simulink model "Solar"  (R2024b)
settings: Solver=VariableStepAuto  StartTime=0.0  StopTime=10.0  RelTol=1e-3
undefined symbols (not defined in the file): sigbuilder_block
libraries: spsSeriesRLCBranchLib x9, spsVoltageMeasurementLib x8, spsDiodeLib x4, spsIGBTLib x1, spsPVArrayLib x1, spsCurrentMeasurementLib x1, spsMosfetLib x1, spsPWMGeneratorDCDCLib x1, sps_lib x1
settings Model: SimulationMode=accelerator  Creator=Jatay  LastModifiedBy=Jatay

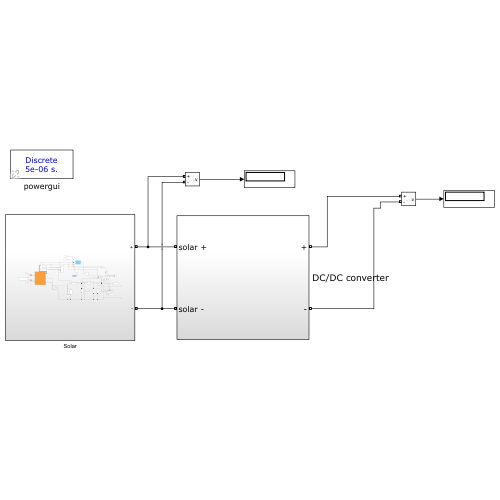
[thumbnail: Simulink's stored preview of the top-level diagram]
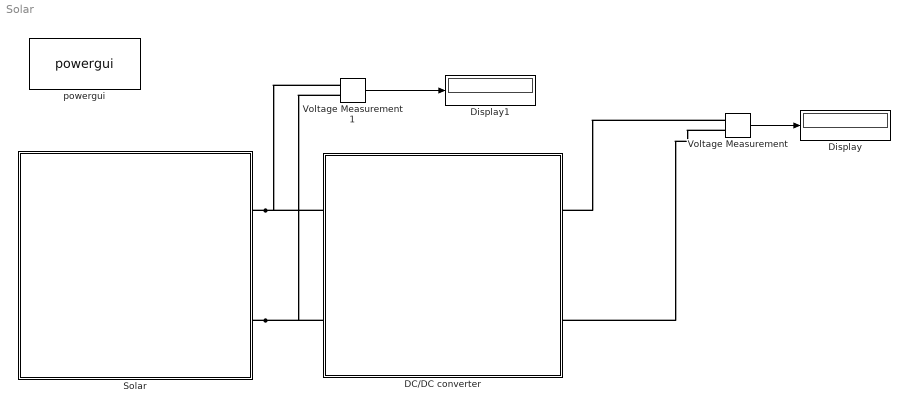
== system Solar ==
  DC/DC converter : Subsystem
  Display : Display
  Display1 : Display
  Solar : Subsystem
  Voltage Measurement : spsVoltageMeasurementLib/Voltage Measurement  PhasorSimulation=off  OutputType=Complex  PSBequivalent=0
  Voltage Measurement1 : spsVoltageMeasurementLib/Voltage Measurement  PhasorSimulation=off  OutputType=Complex  PSBequivalent=0
  powergui : sps_lib/powergui  Priority=1  SimulationMode=Discrete  SampleTime=5e-6  frequency=60  Iterations=50  frequencyindice=0  Pbase=100e6  ErrMax=1e-4  UnitsV=kV  UnitsW=MW  buscounter=0  FunctionMessages=off  echomessages=off  EnableUseOfTLC=off  CurrentSourceSwitches=off  DisableSnubberDevices=off  DisableRonSwitches=off  DisableVfSwitches=off  DisplayEquations=off  AutomaticDiscreteSolvers=off  SolverType=Tustin  Interpol=off  ExternalGateDelay=off  methode=off  Ts=0  x0status=blocks  SPID=off  SwTol=0  HookPort=off  NonlinearTolerance=1e-4  nMaxIteration=100  ContinueOnMaxIteration=off  RestoreLinks=warning  ResistiveCurrentMeasurement=off  Frange=[0:2:500]  Ylog=off  Xlog=on  ShowGrid=off  save=off  variable=ZData  structure=0  ZoomFFT=off  StartTime=0.0  cycles=1  DisplayStyle=1  fundamental=60  FreqAxis=off  MaxFrequency=1000  frequencyindicesteady=1  RmsSteady=1  display=off
  wires:
  Voltage Measurement1/1 -> Display1/1
  Voltage Measurement/1 -> Display/1
  connections:
  Solar/RConn1 -- DC/DC converter/LConn1 -- Voltage Measurement1/LConn1
  Solar/RConn2 -- DC/DC converter/LConn2 -- Voltage Measurement1/LConn2
  Voltage Measurement/LConn2 -- DC/DC converter/RConn2
  Voltage Measurement/LConn1 -- DC/DC converter/RConn1

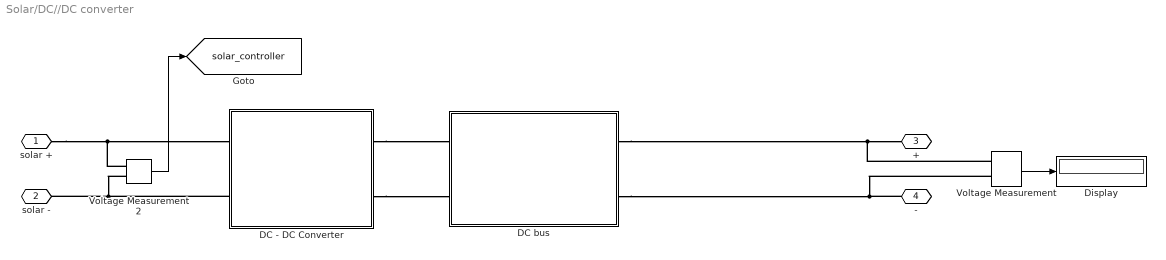
== system Solar/DC//DC converter ==
  DC - DC Converter : Subsystem
  DC bus : Subsystem
  Display : Display
  Voltage Measurement : spsVoltageMeasurementLib/Voltage Measurement  PhasorSimulation=off  OutputType=Complex  PSBequivalent=0
  Voltage Measurement2 : spsVoltageMeasurementLib/Voltage Measurement  PhasorSimulation=off  OutputType=Complex  PSBequivalent=0
  solar + : PMIOPort  Side=Left
  solar - : PMIOPort  Port=2  Side=Left
  + : PMIOPort  Port=3  Side=Right
  - : PMIOPort  Port=4  Side=Right
  tag scope: solar_controller=global
  wires:
  Voltage Measurement2/1 -> [solar_controller]
  Voltage Measurement/1 -> Display/1
  connections:
  DC - DC Converter/RConn1 -- DC bus/LConn1
  solar +/RConn1 -- DC - DC Converter/LConn1 -- Voltage Measurement2/LConn1
  DC - DC Converter/LConn2 -- Voltage Measurement2/LConn2 -- solar -/RConn1
  DC - DC Converter/RConn2 -- DC bus/LConn2
  -/RConn1 -- DC bus/RConn2 -- Voltage Measurement/LConn2
  Voltage Measurement/LConn1 -- DC bus/RConn1 -- +/RConn1

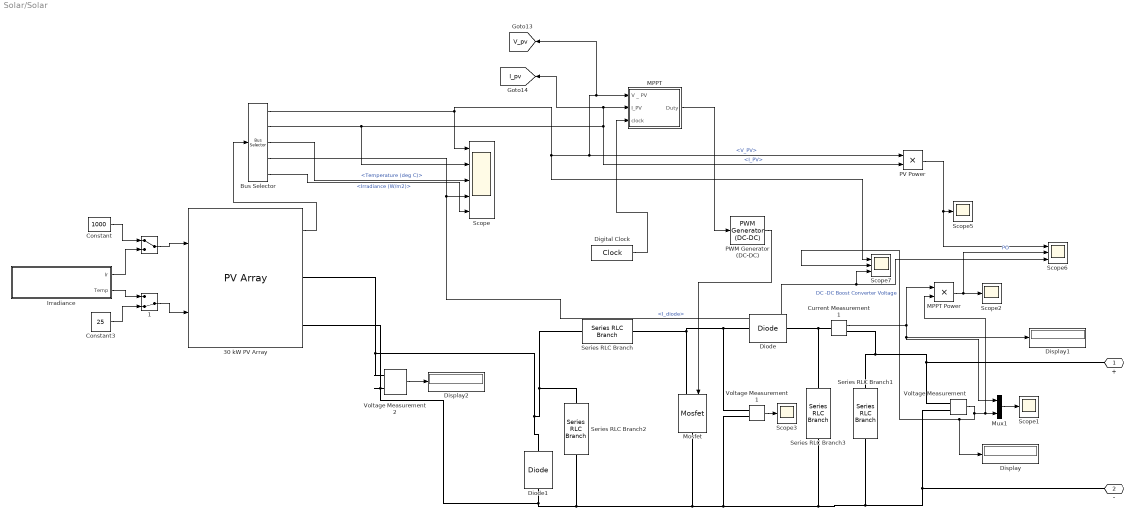
== system Solar/Solar ==
  "      " : ManualSwitch
  "      1" : ManualSwitch  CurrentSetting=0
  30 kW PV Array : spsPVArrayLib/PV Array  Npar=15  Nser=10  PlotType=array @ 1000 W/m2 & specified temperatures  S_vec="[ 1000  500  100 ]"  Temp_C_vec="[ 45 25  ]"  ModuleName=User-defined  PlotWhenSelected=off  Pm=213.15  Ncell=60  Voc=48  Isc=7.84  Vm=29  Im=7.35  beta_Voc_pc=-0.36099  alpha_Isc_pc=0.102  beta_Voc=-0.17328  alpha_Isc=0.0079968  IL=8.2285  I0=2.9956e-10  nI=1.2955  Rsh=7353.5939  Rs=2.0228  RobustModel=off  RobustCellTemperature=25  BAL=on  Tc=1e-6  Tfilter=5e-5
  Bus Selector : BusSelector  OutputSignals=V_PV,I_PV,Temperature (deg C),I_diode,Irradiance (W/m2)
  Constant : Constant  Value=1000
  Constant3 : Constant  Value=25
  Current Measurement1 : spsCurrentMeasurementLib/Current Measurement  PhasorSimulation=off  OutputType=Complex  PSBequivalent=0
  Digital Clock : DigitalClock  SampleTime=0.001
  Diode : spsDiodeLib/Diode  Ron=0.5  Lon=0  Vf=0.7  IC=0  UseSnubber=0  Rs=1e5  Cs=250e-9  Measurements=off
  Diode1 : spsDiodeLib/Diode  Ron=0.5  Lon=0  Vf=0.7  IC=0  UseSnubber=0  Rs=1e5  Cs=250e-9  Measurements=off
  Display : Display
  Display1 : Display
  Display2 : Display
  "Irradiance " : Subsystem  Tag=STV Subsys  LoadFcn=sigbuilder_block('load');  StartFcn=sigbuilder_block('start');  StopFcn=sigbuilder_block('stop');  ClipboardFcn=sigbuilder_block('clipboard');  mask(Sigbuilder block){tuvar=[0:10]}
      mask help: Sigbuilder GUI
      mask init:
      | if ~strcmp(get_param(bdroot(gcbh),'SimulationStatus'),'stopped') tuvar = sigbuilder_block('maskInit'); end
      settings: CopyFcn=sigbuilder_block('copy');  DeleteFcn=sigbuilder_block('delete');  ModelCloseFcn=sigbuilder_block('modelClose');  PreSaveFcn=sigbuilder_block('preSave');  PauseFcn=sigbuilder_block('pause')  ContinueFcn=sigbuilder_block('continue')  NameChangeFcn=sigbuilder_block('namechange');  OpenFcn=sigbuilder_block('open',[5.4 30 1141.2 507.6 ]);  CloseFcn=sigbuilder_block('close');
      mask Display: plot(0, 0, 100, 100,[2, 2, 32, 32, 2], [68, 8, 8, 68, 68],[32, 2], [38, 38], [32, 19, 2],[53, 60, 44], [32, 17, 17, 2],[16, 16, 31, 31]);txt = getActiveGroup(gcbh);text(2, 100, txt,'verticalAlignment', 'top');
  MPPT : Subsystem
  MPPT Power : Product
  Mosfet : spsMosfetLib/Mosfet  Ron=0.1  Lon=0  Rd=0.01  Vfd=0.7  IC=0  Rs=1e5  Cs=inf  Measurements=off
  Mux1 : Mux  Inputs=2
  PV Power : Product
  PWM Generator (DC-DC) : spsPWMGeneratorDCDCLib/PWM Generator (DC-DC)  Fsw=1500  Ts=0
  Scope : Scope  NumInputPorts=5
  Scope{1..3,5} (4 alike) : Scope
  Scope6 : Scope  NumInputPorts=3
  Scope7 : Scope  NumInputPorts=3
  Series RLC Branch : spsSeriesRLCBranchLib/Series RLC Branch  LConnTagsString=__new0  RConnTagsString=__new0  BranchType=L  Resistance=0.001  Inductance=0.4e-1  SetiL0=off  InitialCurrent=0  Capacitance=1e-6  Setx0=off  InitialVoltage=0  Measurements=None
  Series RLC Branch1 : spsSeriesRLCBranchLib/Series RLC Branch  LConnTagsString=__new0  RConnTagsString=__new0  BranchType=R  Resistance=11  Inductance=0.1  SetiL0=off  InitialCurrent=0  Capacitance=100e-6  Setx0=off  InitialVoltage=0  Measurements=None
  Series RLC Branch2 : spsSeriesRLCBranchLib/Series RLC Branch  LConnTagsString=__new0  RConnTagsString=__new0  BranchType=C  Resistance=6  Inductance=0.1  SetiL0=off  InitialCurrent=0  Capacitance=700e-5  Setx0=off  InitialVoltage=0  Measurements=None
  Series RLC Branch3 : spsSeriesRLCBranchLib/Series RLC Branch  LConnTagsString=__new0  RConnTagsString=__new0  BranchType=C  Resistance=6  Inductance=0.1  SetiL0=off  InitialCurrent=0  Capacitance=1000e-5  Setx0=off  InitialVoltage=0  Measurements=None
  Voltage Measurement : spsVoltageMeasurementLib/Voltage Measurement  PhasorSimulation=off  OutputType=Complex  PSBequivalent=0
  Voltage Measurement1 : spsVoltageMeasurementLib/Voltage Measurement  PhasorSimulation=off  OutputType=Complex  PSBequivalent=0
  Voltage Measurement2 : spsVoltageMeasurementLib/Voltage Measurement  PhasorSimulation=off  OutputType=Complex  PSBequivalent=0
  + : PMIOPort  Side=Right
  - : PMIOPort  Port=2  Side=Right
  tag scope: I_pv=global, V_pv=global
  wires:
  Voltage Measurement/1 -> MPPT Power/2, Mux1/2, Display/1, Scope7/2  "DC -DC Boost Converter Voltage"
  PWM Generator (DC-DC)/1 -> Mosfet/1
  Mux1/1 -> Scope1/1
  MPPT Power/1 -> Scope6/2, Scope2/1  "PO"
  Current Measurement1/1 -> MPPT Power/1, Display1/1, Mux1/1
  Voltage Measurement1/1 -> Scope3/1
  Bus Selector/3 -> Scope/3  "<Temperature (deg C)>"
  Bus Selector/4 -> Scope6/3, Scope7/3, Scope/4  "<I_diode>"
  Digital Clock/1 -> MPPT/3(clock)
  MPPT/1(Duty) -> PWM Generator (DC-DC)/1
  PV Power/1 -> Scope6/1, Scope5/1
  "Irradiance "/2(Temp) -> "      1"/1
  Constant3/1 -> "      1"/2
  "Irradiance "/1(Ir) -> "      "/2
  Constant/1 -> "      "/1
  "      "/1 -> 30 kW PV Array/1
  "      1"/1 -> 30 kW PV Array/2
  Voltage Measurement2/1 -> Display2/1
  30 kW PV Array/1 -> Bus Selector/1
  Bus Selector/2 -> Scope/2, MPPT/2(I_PV), [I_pv], PV Power/2  "<I_PV>"
  Bus Selector/5 -> Scope/5  "<Irradiance (W/m2)>"
  Bus Selector/1 -> Scope7/1, PV Power/1, [V_pv], MPPT/1("V _ PV "), Scope/1  "<V_PV>"
  connections:
  Voltage Measurement/LConn2 -- Voltage Measurement2/LConn2 -- 30 kW PV Array/RConn2 -- Diode1/LConn1 -- Series RLC Branch2/RConn1 -- Mosfet/RConn1 -- Voltage Measurement1/LConn2 -- Series RLC Branch3/RConn1 -- Series RLC Branch1/RConn1 -- -/RConn1
  Current Measurement1/RConn1 -- Series RLC Branch1/LConn1 -- Voltage Measurement/LConn1 -- +/RConn1
  Diode/RConn1 -- Series RLC Branch3/LConn1 -- Current Measurement1/LConn1
  Voltage Measurement1/LConn1 -- Series RLC Branch/RConn1 -- Mosfet/LConn1 -- Diode/LConn1
  Series RLC Branch2/LConn1 -- Voltage Measurement2/LConn1 -- 30 kW PV Array/RConn1 -- Diode1/RConn1 -- Series RLC Branch/LConn1

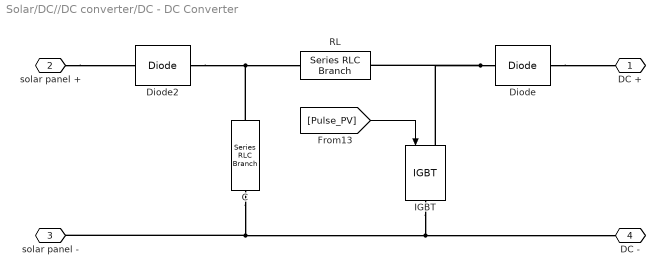
== system Solar/DC//DC converter/DC - DC Converter ==
  C : spsSeriesRLCBranchLib/Series RLC Branch  LConnTagsString=__new0  RConnTagsString=__new0  BranchType=C  Resistance=0.01  Inductance=1e-3  SetiL0=off  InitialCurrent=0  Capacitance=1000e-6  Setx0=on  InitialVoltage=200  Measurements=None
  Diode : spsDiodeLib/Diode  Ron=0.001  Lon=0  Vf=1.1  IC=0  UseSnubber=off  Rs=500  Cs=250e-9  Measurements=off
  Diode2 : spsDiodeLib/Diode  Ron=0.001  Lon=0  Vf=0.7  IC=0  UseSnubber=off  Rs=500  Cs=250e-9  Measurements=off
  IGBT : spsIGBTLib/IGBT  Ron=0.001  Lon=0  Vf=1.1  Tf=1e-6  Tt=2e-6  IC=0  Rs=1e5  Cs=inf  Measurements=off
  RL : spsSeriesRLCBranchLib/Series RLC Branch  LConnTagsString=__new0  RConnTagsString=__new0  BranchType=RL  Resistance=0.05  Inductance=470e-6  SetiL0=off  InitialCurrent=0  Capacitance=1e-6  Setx0=off  InitialVoltage=0  Measurements=None
  DC + : PMIOPort  Side=Right
  solar panel + : PMIOPort  Port=2  Side=Left
  solar panel - : PMIOPort  Port=3  Side=Left
  DC - : PMIOPort  Port=4  Side=Right
  wires:
  [Pulse_PV] -> IGBT/1
  connections:
  Diode/RConn1 -- DC +/RConn1
  Diode2/RConn1 -- C/LConn1 -- RL/LConn1
  Diode/LConn1 -- RL/RConn1 -- IGBT/LConn1
  solar panel +/RConn1 -- Diode2/LConn1
  C/RConn1 -- solar panel -/RConn1 -- DC -/RConn1 -- IGBT/RConn1

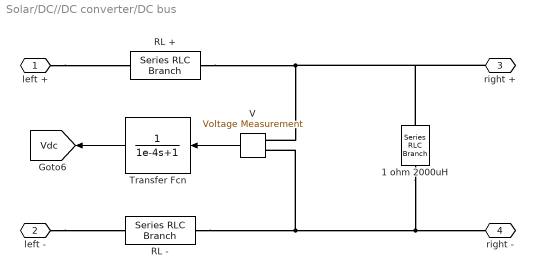
== system Solar/DC//DC converter/DC bus ==
  1 ohm 2000uH : spsSeriesRLCBranchLib/Series RLC Branch  LConnTagsString=__new0  RConnTagsString=__new0  BranchType=RC  Resistance=1  Inductance=0  SetiL0=off  InitialCurrent=0  Capacitance=2000e-6  Setx0=on  InitialVoltage=370  Measurements=None
  RL + : spsSeriesRLCBranchLib/Series RLC Branch  LConnTagsString=__new0  RConnTagsString=__new0  BranchType=RL  Resistance=0.05  Inductance=470e-6  SetiL0=off  InitialCurrent=0  Capacitance=1e-6  Setx0=off  InitialVoltage=0  Measurements=None
  RL - : spsSeriesRLCBranchLib/Series RLC Branch  LConnTagsString=__new0  RConnTagsString=__new0  BranchType=RL  Resistance=0.05  Inductance=470e-6  SetiL0=off  InitialCurrent=0  Capacitance=1e-6  Setx0=off  InitialVoltage=0  Measurements=None
  Transfer Fcn : TransferFcn  Denominator=[1e-4 1]
  V : spsVoltageMeasurementLib/Voltage Measurement  PhasorSimulation=off  OutputType=Complex  PSBequivalent=0
  left + : PMIOPort  Side=Left
  left - : PMIOPort  Port=2  Side=Left
  right + : PMIOPort  Port=3  Side=Right
  right - : PMIOPort  Port=4  Side=Right
  tag scope: Vdc=global
  wires:
  V/1 -> Transfer Fcn/1
  Transfer Fcn/1 -> [Vdc]
  connections:
  RL +/RConn1 -- 1 ohm 2000uH/LConn1 -- right +/RConn1 -- V/LConn1
  RL -/RConn1 -- 1 ohm 2000uH/RConn1 -- right -/RConn1 -- V/LConn2
  left +/RConn1 -- RL +/LConn1
  left -/RConn1 -- RL -/LConn1

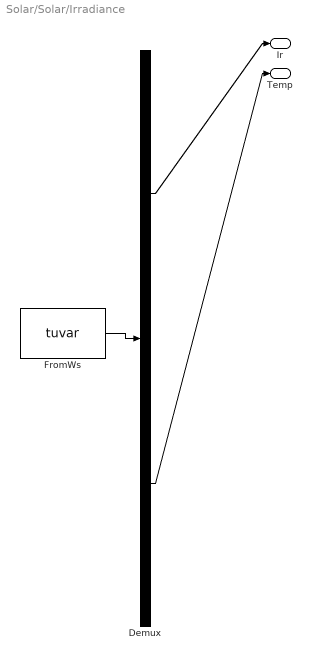
== system Solar/Solar/Irradiance  ==
  Demux : Demux  Tag=STV Demux  Outputs=2
      settings: DisplayOption=none
  FromWs : FromWorkspace  Tag=STV FromWs  VariableName=tuvar
      SigBuilderData=|
      | common.afterFinalStr = 'Extrapolate'
      | common.sampleTime = '0'
      | dataSet(1).timeRange = [0 2]
      | dataSet(1).name = 'Constant Irradiance'
      | dataSet(2).timeRange = [0 2]
      | dataSet(2).name = 'Step Irradiance'
      | dataSet(3).timeRange = [0 1]
      | dataSet(3).name = 'Ramp-up/down Irradiance'
      | sbobj.Groups(1).Name = 'Constant Irradiance'
      | sbobj.Groups(1).Signals(1).Name = 'Ir'
      | sbobj.Groups(1).Signals(1).XData = [0 2]
      | sbobj.Groups(1).Signals(1).YData = [1000 1000]
      | sbobj.Groups(1).Signals(2).Name = 'Temp'
      | sbobj.Groups(1).Signals(2).XData = [0 1 1 2]
      | sbobj.Groups(1).Signals(2).YData = [0 0 1 1]
      | sbobj.Groups(1).TimeRange = [0 2]
      | sbobj.Groups(2).Name = 'Step Irradiance'
      | sbobj.Groups(2).Signals(1).Name = 'Ir'
      | sbobj.Groups(2).Signals(1).XData = [0 0.252 0.252 2]
      | sbobj.Groups(2).Signals(1).YData = [600 600 1000 1000]
      | sbobj.Groups(2).Signals(2).Name = 'Temp'
      | sbobj.Groups(2).Signals(2).XData = [0 1 1 2]
      | sbobj.Groups(2).Signals(2).YData = [0 0 1 1]
      | sbobj.Groups(2).TimeRange = [0 2]
      | sbobj.Groups(3).Name = 'Ramp-up/down Irradiance'
      | sbobj.Groups(3).Signals(1).Name = 'Ir'
      | sbobj.Groups(3).Signals(1).XData = [0 0.3 0.3 0.4 0.4 0.5 0.5 1]
      | sbobj.Groups(3).Signals(1).YData = [1000 1000 800 795 600 600 400 395]
      | sbobj.Groups(3).Signals(2).Name = 'Temp'
      | sbobj.Groups(3).Signals(2).XData = [0 1]
      | sbobj.Groups(3).Signals(2).YData = [25 25]
      | sbobj.Groups(3).TimeRange = [0 1]
  Ir : Outport  Tag=STV Outport
  Temp : Outport  Tag=STV Outport  Port=2
  wires:
  Demux/1 -> Ir/1
  FromWs/1 -> Demux/1
  Demux/2 -> Temp/1

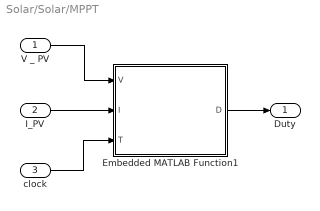
== system Solar/Solar/MPPT ==
  "V _ PV " : Inport
  I_PV : Inport  Port=2
  clock : Inport  Port=3
  Embedded MATLAB Function1 : MATLAB Function  TreatAsAtomicUnit=on
  Duty : Outport  VectorParamsAs1DForOutWhenUnconnected=off
  wires:
  Embedded MATLAB Function1/1(D) -> Duty/1
  clock/1 -> Embedded MATLAB Function1/3(T)
  "V _ PV "/1 -> Embedded MATLAB Function1/1(V)
  I_PV/1 -> Embedded MATLAB Function1/2(I)

== matlab function Solar/MPPT/Embedded MATLAB Function1 ==
  settings: updateMethod=DISCRETE
  data: V input; I input; T input; D output
function D   = PO(V,I,T)
persistent P2  P1  dP d dd n;
if isempty(V)
    V=370;
end
if isempty(I)
    I=0;
end
if isempty(P2)
    P2=0;
end
if isempty(P1)
    P1=0;
end
if isempty(dP)
    dP=0;
end
if isempty(d)
    d=1;
end
if isempty(dd)
    dd=0;
end
if isempty(n)
    n=1;
end
%%%%%%%%%%%%%%%%%%%%%
    if  (T > n*0.02)   %chu ki lay mau 0.02s
    n = n + 1;
    P1=P2;
    P2=V*I;
    dP=P2-P1;
    if (dd==0)
        if dP>1
            dd=0.01;
            d=d+dd;
        else
            if dP<-1
                dd=-0.01;
                d=d+dd;
            else
                dd=0;
            end
        end
    else
        if ((dP<1)&&(dP>-1))
        dd=0;
        d=d+dd;
        else
            if ((dP/dd)>0)
                dd=0.01;
                d=d+dd;
            else
                dd=-0.01;
                d=d+dd;
            end
        end
    end    
    end
D=d/(d+1);
if D<0.4
    D=0.4;
    d=D/(1-D);
else
    if D>0.9
        D=0.9;
        d=D/(1-D);
    else
    end
end
end
